simulink model "CICESE_fric"  (R2021a)
settings: Solver=FixedStepAuto  StartTime=0.0  StopTime=20  FixedStep=1e-4  RelTol=1e-3
libraries: simulink_extras x2
settings Model: Creator=libre  LastModifiedBy=libre

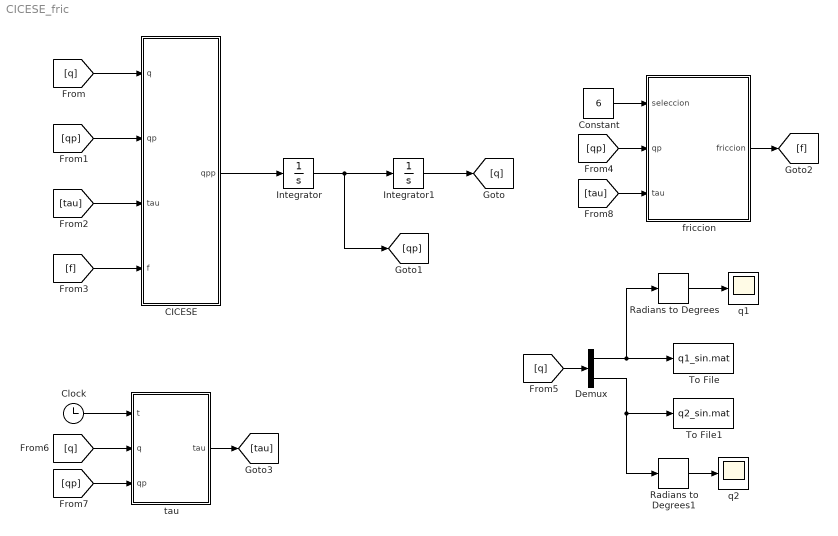
== system CICESE_fric ==
  CICESE : MATLAB Function  TreatAsAtomicUnit=on
  Clock : Clock
  Constant : Constant  Value=6
  Demux : Demux  Outputs=2
  Integrator : Integrator  InitialCondition=[0; 0]
  Integrator1 : Integrator  InitialCondition=[0; 0]
  Radians to Degrees : simulink_extras/Transformations/Radians to Degrees
  Radians to Degrees1 : simulink_extras/Transformations/Radians to Degrees
  To File : ToFile  Filename=q1_sin.mat  SaveFormat=Timeseries
  To File1 : ToFile  Filename=q2_sin.mat  SaveFormat=Timeseries
  friccion : Subsystem
  q1 : Scope
  q2 : Scope
  tau : MATLAB Function  TreatAsAtomicUnit=on
  wires:
  CICESE/1(qpp) -> Integrator/1
  Integrator/1 -> [qp], Integrator1/1
  Integrator1/1 -> [q]
  [q] -> CICESE/1(q)
  [qp] -> CICESE/2(qp)
  [f] -> CICESE/4(f)
  [tau] -> CICESE/3(tau)
  Constant/1 -> friccion/1(seleccion)
  [qp] -> friccion/2(qp)
  friccion/1(friccion) -> [f]
  tau/1(tau) -> [tau]
  Clock/1 -> tau/1(t)
  [q] -> Demux/1
  Demux/1 -> Radians to Degrees/1, To File/1
  Radians to Degrees/1 -> q1/1
  Demux/2 -> Radians to Degrees1/1, To File1/1
  Radians to Degrees1/1 -> q2/1
  [q] -> tau/2(q)
  [qp] -> tau/3(qp)
  [tau] -> friccion/3(tau)

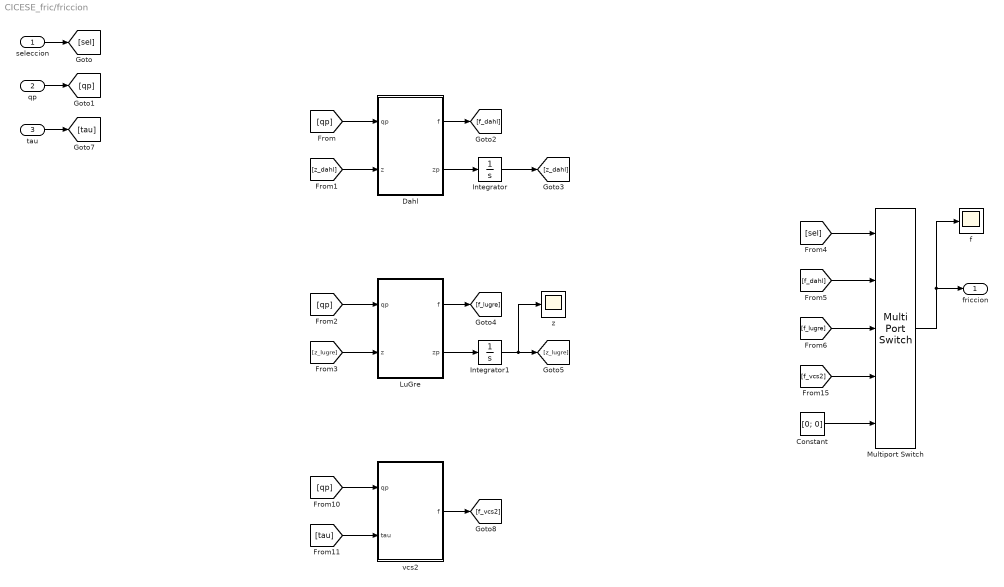
== system CICESE_fric/friccion ==
  seleccion : Inport
  qp : Inport  Port=2
  tau : Inport  Port=3
  Constant : Constant  Value=[0; 0]
  Dahl : MATLAB Function  TreatAsAtomicUnit=on
  Integrator : Integrator  InitialCondition=[0; 0]
  Integrator1 : Integrator  InitialCondition=[0; 0]
  LuGre : MATLAB Function  TreatAsAtomicUnit=on
  Multiport Switch : MultiPortSwitch  Inputs=4
  f : Scope
  vcs2 : MATLAB Function  TreatAsAtomicUnit=on
  z : Scope
  friccion : Outport
  wires:
  seleccion/1 -> [sel]
  qp/1 -> [qp]
  [qp] -> Dahl/1(qp)
  [z_dahl] -> Dahl/2(z)
  Dahl/2(zp) -> Integrator/1
  Dahl/1(f) -> [f_dahl]
  Integrator/1 -> [z_dahl]
  LuGre/2(zp) -> Integrator1/1
  [z_lugre] -> LuGre/2(z)
  LuGre/1(f) -> [f_lugre]
  Integrator1/1 -> z/1, [z_lugre]
  [qp] -> LuGre/1(qp)
  Multiport Switch/1 -> f/1, friccion/1
  [sel] -> Multiport Switch/1
  [f_lugre] -> Multiport Switch/3
  [f_dahl] -> Multiport Switch/2
  tau/1 -> [tau]
  vcs2/1(f) -> [f_vcs2]
  [qp] -> vcs2/1(qp)
  [tau] -> vcs2/2(tau)
  [f_vcs2] -> Multiport Switch/4
  Constant/1 -> Multiport Switch/5

== matlab function CICESE_fric/friccion/Dahl ==
  data: qp input; f output; z input; zp output
function [f,zp] = fcn(qp,z)

sigma_0 = [21418.98; 1013.63];
%%%%%%%%%%%%%%%%%%%%%%%%%%%%%%
sigma_1 = [1404.98; 21.55];
%%%%%%%%%%%%%%%%%%%%%%%%%%%%%%
fc_pos = [12.4401; 1.9181];
fc_neg = [10.9366; 1.7195];
%%%%%%%%%%%%%%%%%%%%%%%%%%%%%%
fs_pos = [10.75; 1.49];
fs_neg = [12.0; 1.45];
%%%%%%%%%%%%%%%%%%%%%%%%%%%%%%
fv_pos = [3.4914; 0.1707];
fv_neg = [2.8016; 0.0839];
%%%%%%%%%%%%%%%%%%%%%%%%%%%%%%
vs_pos = [0.6624*pi/180; 2.697*pi/180];
vs_neg = [0.3687*pi/180; 4.676*pi/180];
%%%%%%%%%%%%%%%%%%%%%%%%%%%%%%
ds_pos = [1.572; 5.281];
ds_neg = [4.625; 3.961];

f = [0; 0];
zp = [0; 0];

for i = 1:2
    if qp(i) > 0 
    f(i) = sigma_0(i)*z(i) + fv_pos(i)*qp(i);
    zp(i) = -sigma_0(i)*abs(qp(i))*z(i)/fc_pos(i) + qp(i);
    else
    f(i) = sigma_0(i)*z(i) + fv_neg(i)*qp(i);
    zp(i) = -sigma_0(i)*abs(qp(i))*z(i)/fc_neg(i) + qp(i);
    end
end

== matlab function CICESE_fric/CICESE ==
  data: q input; qpp output; qp input; tau input; f input
function qpp = fcn(q,qp,tau,f)
g = 9.81;

m11=2.351+0.168*cos(q(2));
m12=0.102+0.084*cos(q(2));
m21=m12;
m22=0.102;

c11=-0.168*sin(q(2))*qp(2);
c12=-0.084*sin(q(2))*qp(2);
c21=0.084*sin(q(2))*qp(1);
c22=0.0;

g1=g*(3.921*sin(q(1))+0.186*sin(q(1) + q(2)));
g2=g*0.186*sin(q(1)+ q(2));

M = [m11 m12; m21 m22];
C = [c11 c12; c21 c22];
g = [g1; g2];

qpp = M\(tau - f - C*qp - g);

== matlab function CICESE_fric/friccion/LuGre ==
  data: qp input; f output; z input; zp output
function [f,zp] = fcn(qp,z)

sigma_0 = [21418.98; 1013.63];
%%%%%%%%%%%%%%%%%%%%%%%%%%%%%%
sigma_1 = [1404.98; 21.55];
%%%%%%%%%%%%%%%%%%%%%%%%%%%%%%
fc_pos = [12.4401; 1.9181];
fc_neg = [10.9366; 1.7195];
%%%%%%%%%%%%%%%%%%%%%%%%%%%%%%
fs_pos = [10.75; 1.49];
fs_neg = [12.0; 1.45];
%%%%%%%%%%%%%%%%%%%%%%%%%%%%%%
fv_pos = [3.4914; 0.1707];
fv_neg = [2.8016; 0.0839];
%%%%%%%%%%%%%%%%%%%%%%%%%%%%%%
vs_pos = [0.6624*pi/180; 2.697*pi/180];
vs_neg = [0.3687*pi/180; 4.676*pi/180];
%%%%%%%%%%%%%%%%%%%%%%%%%%%%%%
ds_pos = [1.572; 5.281];
ds_neg = [4.625; 3.961];


f = [0; 0];
zp = [0; 0];

for i = 1:2
    if qp(i) > 0 
    g = fc_pos(i) + (fs_pos(i) - fc_pos(i))*exp(-abs(qp(i)/vs_pos(i))^ds_pos(i));    
    zp(i) = -sigma_0(i)*abs(qp(i))*z(i)/g + qp(i);
    f(i) = sigma_0(i)*z(i) + sigma_1(i)*zp(i) + fv_pos(i)*qp(i);
    else
    g = fc_neg(i) + (fs_neg(i) - fc_neg(i))*exp(-abs(qp(i)/vs_neg(i))^ds_neg(i));
    zp(i) = -sigma_0(i)*abs(qp(i))*z(i)/g + qp(i);
    f(i) = sigma_0(i)*z(i) + sigma_1(i)*zp(i) + fv_neg(i)*qp(i);
    end
end

== matlab function CICESE_fric/tau ==
  data: t input; tau output; q input; qp input
function tau = fcn(t,q,qp)


% g = 9.81;
% kp1 = 50.0; 
% kp2 = 3.0;
% kv1 = 1.0*180/pi;
% kv2 = 0.01*180/pi;
% lambda1 = 2.288*180/pi;
% lambda2 = 0.175*180/pi;
% 
% g1 = g*(3.921*sin(q(1))+0.186*sin(q(1) + q(2)));
% g2 = g*0.186*sin(q(1) + q(2));
% 
% if art == 1
%     tau = [0.5*t; kp2*tanh(lambda2*(-q(2))) - kv2*qp(2) + g2];
% elseif art == 2
%     tau = [kp1*tanh(lambda1*(-q(1))) - kv1*qp(1) + g1; 0.1*t];    
% else
%     tau = [0; 0];
% end

tau = [20; -2]*sin(2*pi*t*0.1);

== matlab function CICESE_fric/friccion/vcs2 ==
  data: qp input; f output; tau input
function f = fcn(qp,tau)

sigma_0 = [21418.98; 1013.63];
%%%%%%%%%%%%%%%%%%%%%%%%%%%%%%
sigma_1 = [1404.98; 21.55];
%%%%%%%%%%%%%%%%%%%%%%%%%%%%%%
fc_pos = [12.4401; 1.9181];
fc_neg = [10.9366; 1.7195];
%%%%%%%%%%%%%%%%%%%%%%%%%%%%%%
fs_pos = [10.75; 1.49];
fs_neg = [12.0; 1.45];
%%%%%%%%%%%%%%%%%%%%%%%%%%%%%%
fv_pos = [3.4914; 0.1707];
fv_neg = [2.8016; 0.0839];
%%%%%%%%%%%%%%%%%%%%%%%%%%%%%%
vs_pos = [0.6624*pi/180; 2.697*pi/180];
vs_neg = [0.3687*pi/180; 4.676*pi/180];
%%%%%%%%%%%%%%%%%%%%%%%%%%%%%%
ds_pos = [1.572; 5.281];
ds_neg = [4.625; 3.961];
f = [0; 0];

for i = 1:2
    if qp(i) > 0 
        f(i) = fc_pos(i) + (fs_pos(i) - fc_pos(i))*exp(-abs(qp(i)/vs_pos(i))^ds_pos(i)) + fv_pos(i)*qp(i);
    elseif qp(i) < 0
        f(i) = fc_neg(i) + (fs_neg(i) - fc_neg(i))*exp(-abs(qp(i)/vs_neg(i))^ds_neg(i)) + fv_neg(i)*qp(i);
    else
        if tau(i) > fs_pos(i)
            f(i) = fs_pos(i);
        elseif tau(i) < fs_neg(i)
            f(i) = fs_neg(i);
        else
           f(i) = tau(i);
        end
    end
end
